simulink model "upsample_tut1"  (Simulink 5.0)
settings: Solver=FixedStepDiscrete  SolverMode=SingleTasking  StartTime=0.0  StopTime=5  RelTol=1e-3
libraries: dspsigattribs x1, dspsrcs4 x1, dspsigops x1
settings Model: Creator=ckamachi  LastModifiedBy=ckamachi  ExtModeTrigMode=oneshot  ExtModeArmWhenConnect=off  LimitDataPoints=off  BlockReductionOpt=off  BooleanDataType=off

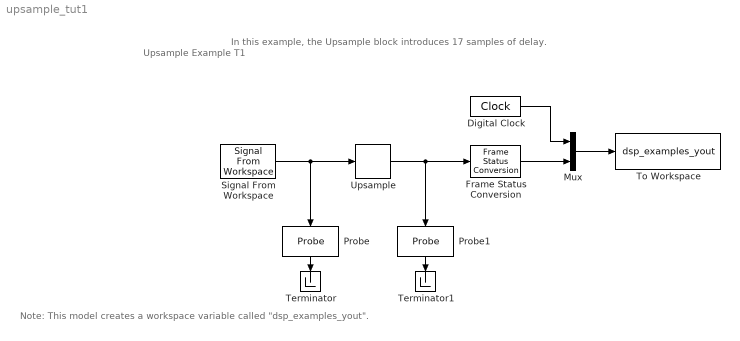
== system upsample_tut1 ==
  note: Upsample Example T1
  note: In this example, the Upsample block introduces 17 samples of delay.
  note: Note: This model creates a workspace variable called "dsp_examples_yout".
  Digital Clock : DigitalClock  SampleTime=1/4
  Frame Status Conversion : dspsigattribs/Frame Status Conversion  growRefPort=off  outframe=Sample-based
  Mux : Mux  Inputs=2
  Probe : Probe  Orientation=down  ProbeWidth=off  ProbeComplexSignal=off
  Probe1 : Probe  Orientation=down  ProbeWidth=off  ProbeComplexSignal=off
  Signal From Workspace : dspsrcs4/Signal From Workspace  X=1:100  Ts=1/4  nsamps=4  OutputAfterFinalValue=Setting to zero
  Terminator : Terminator
      settings: Orientation=down
  Terminator1 : Terminator
      settings: Orientation=down
  To Workspace : ToWorkspace  VariableName=dsp_examples_yout  SampleTime=-1  SaveFormat=Array
  Upsample : dspsigops/Upsample  N=4  phase=0  ic=-1  mode=Maintain input frame size
  wires:
  Mux/1 -> To Workspace/1
  Digital Clock/1 -> Mux/1
  Signal From Workspace/1 -> Upsample/1, Probe/1
  Upsample/1 -> Probe1/1, Frame Status Conversion/1
  Frame Status Conversion/1 -> Mux/2
  Probe/1 -> Terminator/1
  Probe1/1 -> Terminator1/1
